simulink library "INT_CoETM_ClgDem"  (R2016b)
settings: Solver=VariableStepAuto  StartTime=0.0  StopTime=10.0  RelTol=1e-3
settings Model: Creator=xinchangran  LastModifiedBy=xinchangran

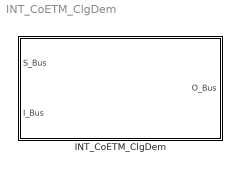
== system INT_CoETM_ClgDem ==
  INT_CoETM_ClgDem : Subsystem

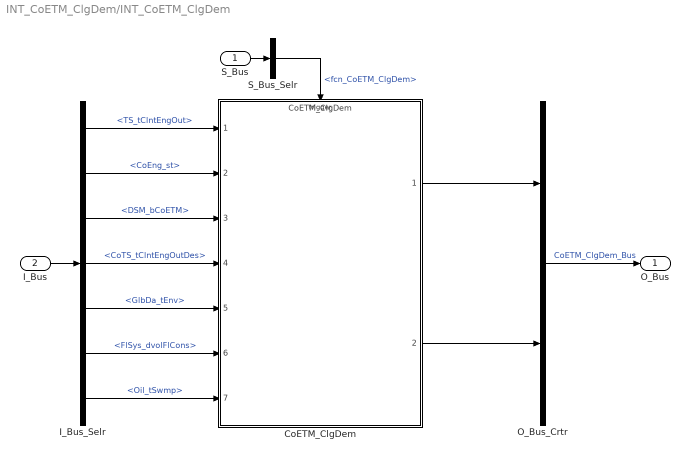
== system INT_CoETM_ClgDem/INT_CoETM_ClgDem ==
  S_Bus : Inport
  I_Bus : Inport  Port=2
  CoETM_ClgDem : ModelReference  ModelNameDialog=CoETM_ClgDem  SimulationMode=Normal  ModelReferenceVersion=1.162  TriggerPortName=function  TriggerPortTriggerType=function-call  TriggerPortStatesWhenEnabling=held
  I_Bus_Selr : BusSelector  OutputSignals=TS_tClntEngOut,CoEng_st,DSM_bCoETM,CoTS_tClntEngOutDes,GlbDa_tEnv,FlSys_dvolFlCons,Oil_tSwmp
  O_Bus_Crtr : BusCreator  Inputs=2
  S_Bus_Selr : BusSelector  OutputSignals=fcn_CoETM_ClgDem
  O_Bus : Outport
  wires:
  S_Bus_Selr/1 -> CoETM_ClgDem/Trigger  "<fcn_CoETM_ClgDem>"
  S_Bus/1 -> S_Bus_Selr/1
  I_Bus/1 -> I_Bus_Selr/1
  I_Bus_Selr/1 -> CoETM_ClgDem/1  "<TS_tClntEngOut>"
  I_Bus_Selr/2 -> CoETM_ClgDem/2  "<CoEng_st>"
  I_Bus_Selr/3 -> CoETM_ClgDem/3  "<DSM_bCoETM>"
  I_Bus_Selr/4 -> CoETM_ClgDem/4  "<CoTS_tClntEngOutDes>"
  I_Bus_Selr/5 -> CoETM_ClgDem/5  "<GlbDa_tEnv>"
  I_Bus_Selr/6 -> CoETM_ClgDem/6  "<FlSys_dvolFlCons>"
  I_Bus_Selr/7 -> CoETM_ClgDem/7  "<Oil_tSwmp>"
  O_Bus_Crtr/1 -> O_Bus/1  "CoETM_ClgDem_Bus"
  CoETM_ClgDem/1 -> O_Bus_Crtr/1
  CoETM_ClgDem/2 -> O_Bus_Crtr/2
